simulink model "lab4_PID"  (Simulink 10.1)
settings: Solver=ode3  StartTime=0.0  StopTime=inf  FixedStep=.01  RelTol=1e-3  EnableMultiTasking=on
undefined symbols (not defined in the file): Serial_Port, Standard_Devices
libraries: rtwinlib x2, simulink x2, sldrtlib x2
settings Model: Creator=Jenna Toennies  LastModifiedBy=hp  SimulationMode=external
settings DataIOCC: LimitDataPoints=on  SignalLoggingSaveFormat=ModelDataLogs
settings OptimizationCC: ExpressionDepthLimit=2147483647
settings DebuggingCC: SolverPrmCheckMsg=warning  FcnCallInpInsideContextMsg=warning  StateNameClashWarn=warning
settings HardwareCC: ProdIntDivRoundTo=Zero  ProdEndianess=LittleEndian  ProdHWDeviceType=Generic->32-bit x86 compatible
settings SFSimCC: SimParseCustomCode=off
settings RTWCC: Description=Real-Time Windows Target  SystemTargetFile=rtwin.tlc  TemplateMakefile=rtwin.tmf  RTWCompilerOptimization=on
settings CodeAppCC: MaxIdLength=95
settings TargetCC: TargetLibSuffix=_rtwin.lib  TargetPreCompLibLocation=C:\Program Files\MATLAB\R2010a\toolbox\rtw\targets\rtwin\lib

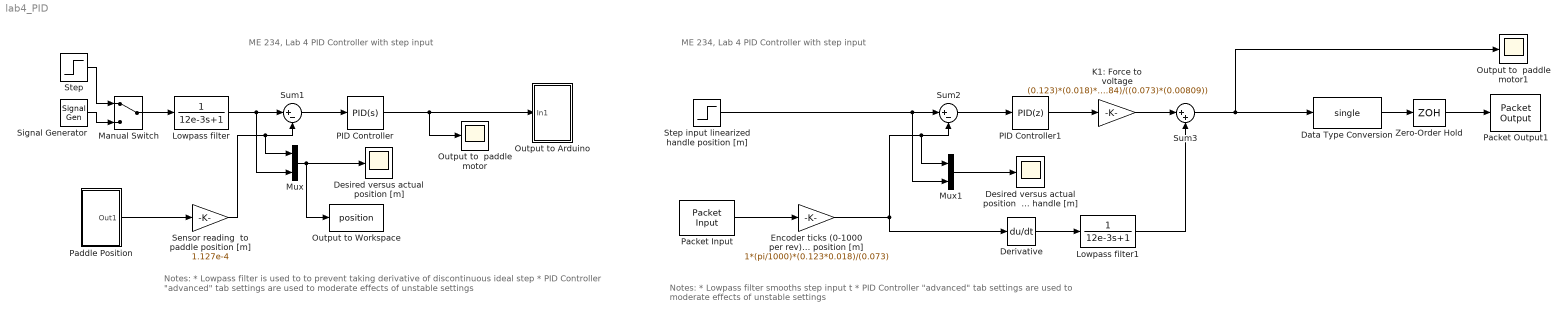
== system lab4_PID ==
  note: ME 234, Lab 4
      | PID Controller with step input
  note: Notes:
      | * Lowpass filter is used to to prevent taking derivative of discontinuous ideal step
      | * PID Controller "advanced" tab settings are used to moderate effects of unstable settings
  note: ME 234, Lab 4
      | PID Controller with step input
  note: Notes:
      | * Lowpass filter smooths step input t
      | * PID Controller "advanced" tab settings are used to moderate effects of unstable settings
  Data Type Conversion : DataTypeConversion  OutDataTypeStr=single
  Derivative : Derivative
  Desired versus actual position  of paddle handle [m] : Scope
  Desired versus actual position [m] : Scope
  "Encoder ticks (0-1000 per rev)  to paddle position [m] " : Gain  Gain=1*(pi/1000)*(0.123*0.018)/(0.073)  OutDataTypeStr=double
  K1: Force to voltage : Gain  Gain=(0.123)*(0.018)*(1.84)/((0.073)*(0.00809))  OutDataTypeStr=double
  Lowpass filter : TransferFcn  Denominator=[12e-3 1]
  Lowpass filter1 : TransferFcn  Denominator=[12e-3 1]
  Manual Switch : ManualSwitch
  Mux : Mux  Inputs=2
  Mux1 : Mux  Inputs=2
  Output to  paddle motor : Scope
  Output to  paddle motor1 : Scope
  Output to Arduino : Subsystem
  Output to Workspace : ToWorkspace  VariableName=position  SampleTime=-1
  PID Controller : simulink/Continuous/PID Controller  Controller=PID  Form=Parallel  TimeDomain=Continuous-time  UseExternalTs=off  SampleTime=0.01  IntegratorMethod=Forward Euler  FilterMethod=Forward Euler  ControllerParametersSource=internal  P=5  I=0  D=1  UseFilter=on  N=100  TunerSelectOption=Transfer Function Based (PID Tuner App)  InitialConditionSource=internal  InitialConditionForIntegrator=0  InitialConditionForFilter=0  DifferentiatorICPrevScaledInput=0  ExternalReset=none  TrackingMode=off  Kt=1  LimitOutput=on  UpperSaturationLimit=1  LowerSaturationLimit=-1  LinearizeAsGain=off  AntiWindupMode=clamping  Kb=1  POutMin=[]  POutMax=[]  IOutMin=[]  IOutMax=[]  DOutMin=[]  DOutMax=[]  NOutMin=[]  NOutMax=[]  SumOutMin=[]  SumOutMax=[]  SaturationOutMin=[]  SaturationOutMax=[]  PParamMin=[]  PParamMax=[]  IParamMin=[]  IParamMax=[]  DParamMin=[]  DParamMax=[]  NParamMin=[]  NParamMax=[]  KbParamMin=[]  KbParamMax=[]  KtParamMin=[]  KtParamMax=[]  KbOutMin=[]  KbOutMax=[]  KtOutMin=[]  KtOutMax=[]  IntegratorOutMin=[]  IntegratorOutMax=[]  FilterOutMin=[]  FilterOutMax=[]  SumI1OutMin=[]  SumI1OutMax=[]  SumI2OutMin=[]  SumI2OutMax=[]  SumI3OutMin=[]  SumI3OutMax=[]  SumI4OutMin=[]  SumI4OutMax=[]  SumDOutMin=[]  SumDOutMax=[]  DifferentiatorOutMin=[]  DifferentiatorOutMax=[]  FilterDiffOutCoefMin=[]  FilterDiffOutCoefMax=[]  ReciprocalOutMin=[]  ReciprocalOutMax=[]  SumDenOutMin=[]  SumDenOutMax=[]  SumNumOutMin=[]  SumNumOutMax=[]  DivideOutMin=[]  DivideOutMax=[]  UdiffTsProdOutMin=[]  UdiffTsProdOutMax=[]  NTsProdOutMin=[]  NTsProdOutMax=[]  UintegralTsProdOutMin=[]  UintegralTsProdOutMax=[]  UngainTsProdOutMin=[]  UngainTsProdOutMax=[]  IntegratorContinuousStateAttributes=''  IntegratorStateMustResolveToSignalObject=off  IntegratorRTWStateStorageClass=Auto  FilterContinuousStateAttributes=''  FilterStateMustResolveToSignalObject=off  FilterRTWStateStorageClass=Auto  ParallelPVariant=InternalParameters  IdealPVariant=Disabled  IVariant=InternalParameters  DVariant=InternalParameters  IntegratorVariant=Continuous  SatVariant=Enabled  AWVariant=ContClampingParallel  PCopyVariant=Disabled  TRVariant=Disabled  FdbkBlocksVariant=Forward  IdealPFdbkVariant=Disabled  SatFdbkVariant=Disabled  DerivativeFilterVariant=ContFilter  NVariant=InternalParameters  NCopyVariant=Disabled  FilterICVariant=InternalICsFilter  IntegratorICVariant=InternalICs  ExternalResetVariant=Disabled  TRSumVariant=Passthrough  SumFdbkVariant=Disabled  SumVariant=Sum_PID  TsampFilterVariant=InternalTs  TsampNgainVariant=Passthrough  TsampIntegralVariant=Passthrough
  PID Controller1 : simulink/Continuous/PID Controller  Controller=PID  Form=Ideal  TimeDomain=Discrete-time  UseExternalTs=off  SampleTime=0.008  IntegratorMethod=Forward Euler  FilterMethod=Forward Euler  ControllerParametersSource=internal  P=30  I=0  D=0.02  UseFilter=on  N=25  TunerSelectOption=Transfer Function Based (PID Tuner App)  InitialConditionSource=internal  InitialConditionForIntegrator=0  InitialConditionForFilter=0  DifferentiatorICPrevScaledInput=0  ExternalReset=none  TrackingMode=off  Kt=1  LimitOutput=off  UpperSaturationLimit=2  LowerSaturationLimit=-2  LinearizeAsGain=off  AntiWindupMode=clamping  Kb=1  POutMin=[]  POutMax=[]  IOutMin=[]  IOutMax=[]  DOutMin=[]  DOutMax=[]  NOutMin=[]  NOutMax=[]  SumOutMin=[]  SumOutMax=[]  SaturationOutMin=[]  SaturationOutMax=[]  PParamMin=[]  PParamMax=[]  IParamMin=[]  IParamMax=[]  DParamMin=[]  DParamMax=[]  NParamMin=[]  NParamMax=[]  KbParamMin=[]  KbParamMax=[]  KtParamMin=[]  KtParamMax=[]  KbOutMin=[]  KbOutMax=[]  KtOutMin=[]  KtOutMax=[]  IntegratorOutMin=[]  IntegratorOutMax=[]  FilterOutMin=[]  FilterOutMax=[]  SumI1OutMin=[]  SumI1OutMax=[]  SumI2OutMin=[]  SumI2OutMax=[]  SumI3OutMin=[]  SumI3OutMax=[]  SumI4OutMin=[]  SumI4OutMax=[]  SumDOutMin=[]  SumDOutMax=[]  DifferentiatorOutMin=[]  DifferentiatorOutMax=[]  FilterDiffOutCoefMin=[]  FilterDiffOutCoefMax=[]  ReciprocalOutMin=[]  ReciprocalOutMax=[]  SumDenOutMin=[]  SumDenOutMax=[]  SumNumOutMin=[]  SumNumOutMax=[]  DivideOutMin=[]  DivideOutMax=[]  UdiffTsProdOutMin=[]  UdiffTsProdOutMax=[]  NTsProdOutMin=[]  NTsProdOutMax=[]  UintegralTsProdOutMin=[]  UintegralTsProdOutMax=[]  UngainTsProdOutMin=[]  UngainTsProdOutMax=[]  IntegratorContinuousStateAttributes=''  IntegratorStateMustResolveToSignalObject=off  IntegratorRTWStateStorageClass=Auto  FilterContinuousStateAttributes=''  FilterStateMustResolveToSignalObject=off  FilterRTWStateStorageClass=Auto  ParallelPVariant=Passthrough  IdealPVariant=InternalParameters  IVariant=InternalParameters  DVariant=InternalParameters  IntegratorVariant=Discrete  SatVariant=Disabled  AWVariant=Passthrough  PCopyVariant=Disabled  TRVariant=Disabled  FdbkBlocksVariant=Forward  IdealPFdbkVariant=Disabled  SatFdbkVariant=Disabled  DerivativeFilterVariant=ForwardEulerFilter  NVariant=InternalParameters  NCopyVariant=Disabled  FilterICVariant=InternalICsFilter  IntegratorICVariant=InternalICs  ExternalResetVariant=Disabled  TRSumVariant=Passthrough  SumFdbkVariant=Disabled  SumVariant=Sum_PID  TsampFilterVariant=InternalTs  TsampNgainVariant=Passthrough  TsampIntegralVariant=Passthrough
  Packet Input : sldrtlib/Packet Input  SampleTime=.008  MaxMissedTicks=10  ShowMissedTicks=off  YieldWhenWaiting=off  DrvName=Standard_Devices/Serial_Port  DrvAddress=9  DrvOptions=[115200 8 0 0 0 0 0]  PacketSize=4  DataTypes='1*int32'  ShowReady=off  ShowError=off  PacketID=1  ByteOrder=1  ShowTimestamp=off
      settings: AttributesFormatString=Standard Devices\nSerial Port [9h]
  Packet Output1 : sldrtlib/Packet Output  SampleTime=.008  MaxMissedTicks=10  ShowMissedTicks=off  YieldWhenWaiting=off  DrvName=Standard_Devices/Serial_Port  DrvAddress=9  DrvOptions=[115200 8 0 0 0 0 0]  PacketSize=4  DataTypes='1*single'  ShowReady=off  ShowError=off  PacketID=1  ByteOrder=1  InitialValue=[]  FinalValue=[]
      settings: AttributesFormatString=Standard Devices\nSerial Port [9h]
  Paddle Position : Subsystem
  "Sensor reading  to paddle position [m] " : Gain  Gain=1.127e-4  OutDataTypeStr=double
  Signal Generator : SignalGenerator  WaveForm=square  Amplitude=0.04  Frequency=3  Units=rad/sec
  Step : Step  SampleTime=0
  Step input linearized handle position [m] : Step  Time=2  After=0.05  SampleTime=0.008
  Sum1 : Sum  Inputs=|+-
  Sum2 : Sum  Inputs=|+-
  Sum3 : Sum  Inputs=|++
  Zero-Order Hold : ZeroOrderHold  SampleTime=.008
  wires:
  Paddle Position/1(Out1) -> "Sensor reading  to paddle position [m] "/1
  PID Controller/1 -> Output to  paddle motor/1, Output to Arduino/1(In1)
  "Sensor reading  to paddle position [m] "/1 -> Sum1/2, Mux/1
  Mux/1 -> Desired versus actual position [m]/1, Output to Workspace/1
  Lowpass filter/1 -> Sum1/1, Mux/2
  Sum1/1 -> PID Controller/1
  Manual Switch/1 -> Lowpass filter/1
  Signal Generator/1 -> Manual Switch/2
  Step/1 -> Manual Switch/1
  K1: Force to voltage/1 -> Sum3/1
  Derivative/1 -> Lowpass filter1/1
  PID Controller1/1 -> K1: Force to voltage/1
  Sum3/1 -> Data Type Conversion/1, Output to  paddle motor1/1
  Packet Input/1 -> "Encoder ticks (0-1000 per rev)  to paddle position [m] "/1
  Step input linearized handle position [m]/1 -> Sum2/1, Mux1/2
  Mux1/1 -> Desired versus actual position  of paddle handle [m]/1
  Data Type Conversion/1 -> Zero-Order Hold/1
  Zero-Order Hold/1 -> Packet Output1/1
  "Encoder ticks (0-1000 per rev)  to paddle position [m] "/1 -> Sum2/2, Mux1/1, Derivative/1
  Sum2/1 -> PID Controller1/1
  Lowpass filter1/1 -> Sum3/2

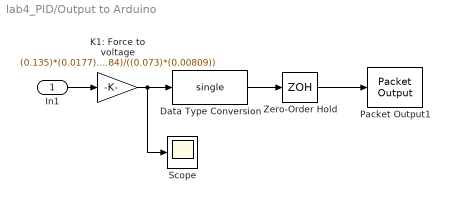
== system lab4_PID/Output to Arduino ==
  In1 : Inport
  Data Type Conversion : DataTypeConversion  OutDataTypeStr=single
  K1: Force to voltage : Gain  Gain=(0.135)*(0.0177)*(1.84)/((0.073)*(0.00809))  OutDataTypeStr=double
  Packet Output1 : rtwinlib/Packet Output  SampleTime=0.01  DrvName=Standard_Devices/Serial_Port  DrvAddress=7  DrvOptions=[115200 8 0 0 0 0 0 0]  PacketSize=4  DataTypes='1*single'  ShowReady=off  ShowError=off  PacketID=1  InitialValue=[]  FinalValue=[]
      settings: AttributesFormatString=Standard Devices\nSerial Port [7h]  SourceProductBaseCode=WT
  Scope : Scope
  Zero-Order Hold : ZeroOrderHold  SampleTime=0.01
  wires:
  Data Type Conversion/1 -> Zero-Order Hold/1
  Zero-Order Hold/1 -> Packet Output1/1
  In1/1 -> K1: Force to voltage/1
  K1: Force to voltage/1 -> Data Type Conversion/1, Scope/1

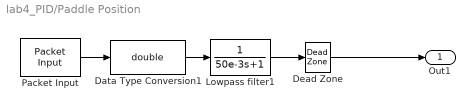
== system lab4_PID/Paddle Position ==
  Data Type Conversion1 : DataTypeConversion  OutDataTypeStr=double
  Dead Zone : DeadZone  LowerValue=499.5  UpperValue=500.5  SaturateOnIntegerOverflow=on
  Lowpass filter1 : TransferFcn  Denominator=[50e-3 1]
  Packet Input : rtwinlib/Packet Input  SampleTime=.01  DrvName=Standard_Devices/Serial_Port  DrvAddress=7  DrvOptions=[115200 8 0 0 0 0 0 0]  PacketSize=2  DataTypes='1*int16'  ShowReady=off  ShowError=off  PacketID=1  ShowTimestamp=off
      settings: AttributesFormatString=Standard Devices\nSerial Port [7h]  SourceProductBaseCode=WT
  Out1 : Outport
  wires:
  Packet Input/1 -> Data Type Conversion1/1
  Dead Zone/1 -> Out1/1
  Data Type Conversion1/1 -> Lowpass filter1/1
  Lowpass filter1/1 -> Dead Zone/1
